simulink model "ap_12B_cocoSim_pp"  (Simulink 8.5)
settings: Solver=ode3  StartTime=0.0  StopTime=100  FixedStep=Ts  RelTol=1e-3
undefined symbols (not defined in the file): beaver_b, beaver_c, beaver_mass, beaver_S, Cl0, Cl_alpha2_dpt, Cl_beta, Cl_da, Cl_da_alpha, Cl_dr, Cl_p, Cl_r, Cm0, Cm_alpha, Cm_alpha2, Cm_beta2, Cm_de, Cm_df, Cm_dpt, Cm_q, Cm_r, Cn0, Cn_beta, Cn_beta3, Cn_da, Cn_dpt3, Cn_dr, Cn_p, Cn_q, Cn_r, Cx0, Cx_alpha, Cx_alpha2, Cx_alpha3, Cx_df, Cx_df_alpha, Cx_dpt, Cx_dpt2_alpha, Cx_dr, Cx_q, Cy0, Cy_beta, Cy_da, Cy_dr, Cy_dr_alpha, Cy_p, Cy_r, Cz0, Cz_alpha, Cz_alpha3, Cz_de, Cz_de_beta, Cz_df, Cz_df_alpha, Cz_dpt, Cz_q, d2r, fin_act_1, fin_act_2, fin_act_3 ... (+23)
libraries: simulink x12, aerolibtransform2 x9, aerolibutil x7, aerolibasang x7, aerolibadynsys x3, aerolib6dofsys x2, aerolib6dof2 x1
(part 3 of 3)

== system ap_12B_cocoSim_pp/Autopilot/Pitch_Autopilot/Altitude Mode/Lookup Table_pp/Interpolate5 ==
  InportIn : Inport
  InportIdx1 : Inport  Port=2
  InportIdx2 : Inport  Port=3
  InportData1 : Inport  Port=4
  InportData2 : Inport  Port=5
  Interpolate : Product  Inputs=*/*  SaturateOnIntegerOverflow=on  RndMeth=Zero  InputSameDT=on  OutDataTypeStr=Inherit: Same as first input
  Sum1 : Sum  Inputs=+-  SaturateOnIntegerOverflow=on  InputSameDT=on  OutDataTypeStr=Inherit: Same as first input
  Sum2 : Sum  Inputs=-+  SaturateOnIntegerOverflow=on  InputSameDT=on  OutDataTypeStr=Inherit: Same as first input
  Sum3 : Sum  Inputs=-+  SaturateOnIntegerOverflow=on  InputSameDT=on  OutDataTypeStr=Inherit: Same as first input
  Sum4 : Sum  SaturateOnIntegerOverflow=on  InputSameDT=on  OutDataTypeStr=Inherit: Same as first input
  Out : Outport
  wires:
  InportIn/1 -> Sum1/1
  InportIdx1/1 -> Sum1/2, Sum2/1
  InportIdx2/1 -> Sum2/2
  InportData1/1 -> Sum3/1, Sum4/2
  InportData2/1 -> Sum3/2
  Sum1/1 -> Interpolate/1
  Sum2/1 -> Interpolate/2
  Sum3/1 -> Interpolate/3
  Interpolate/1 -> Sum4/1
  Sum4/1 -> Out/1

== system ap_12B_cocoSim_pp/Autopilot/Pitch_Autopilot/Altitude Mode/Lookup Table_pp/Interpolate6 ==
  InportIn : Inport
  InportIdx1 : Inport  Port=2
  InportIdx2 : Inport  Port=3
  InportData1 : Inport  Port=4
  InportData2 : Inport  Port=5
  Interpolate : Product  Inputs=*/*  SaturateOnIntegerOverflow=on  RndMeth=Zero  InputSameDT=on  OutDataTypeStr=Inherit: Same as first input
  Sum1 : Sum  Inputs=+-  SaturateOnIntegerOverflow=on  InputSameDT=on  OutDataTypeStr=Inherit: Same as first input
  Sum2 : Sum  Inputs=-+  SaturateOnIntegerOverflow=on  InputSameDT=on  OutDataTypeStr=Inherit: Same as first input
  Sum3 : Sum  Inputs=-+  SaturateOnIntegerOverflow=on  InputSameDT=on  OutDataTypeStr=Inherit: Same as first input
  Sum4 : Sum  SaturateOnIntegerOverflow=on  InputSameDT=on  OutDataTypeStr=Inherit: Same as first input
  Out : Outport
  wires:
  InportIn/1 -> Sum1/1
  InportIdx1/1 -> Sum1/2, Sum2/1
  InportIdx2/1 -> Sum2/2
  InportData1/1 -> Sum3/1, Sum4/2
  InportData2/1 -> Sum3/2
  Sum1/1 -> Interpolate/1
  Sum2/1 -> Interpolate/2
  Sum3/1 -> Interpolate/3
  Interpolate/1 -> Sum4/1
  Sum4/1 -> Out/1

== system ap_12B_cocoSim_pp/Autopilot/Pitch_Autopilot/Altitude Mode/Lookup Table_pp/Interpolate7 ==
  InportIn : Inport
  InportIdx1 : Inport  Port=2
  InportIdx2 : Inport  Port=3
  InportData1 : Inport  Port=4
  InportData2 : Inport  Port=5
  Interpolate : Product  Inputs=*/*  SaturateOnIntegerOverflow=on  RndMeth=Zero  InputSameDT=on  OutDataTypeStr=Inherit: Same as first input
  Sum1 : Sum  Inputs=+-  SaturateOnIntegerOverflow=on  InputSameDT=on  OutDataTypeStr=Inherit: Same as first input
  Sum2 : Sum  Inputs=-+  SaturateOnIntegerOverflow=on  InputSameDT=on  OutDataTypeStr=Inherit: Same as first input
  Sum3 : Sum  Inputs=-+  SaturateOnIntegerOverflow=on  InputSameDT=on  OutDataTypeStr=Inherit: Same as first input
  Sum4 : Sum  SaturateOnIntegerOverflow=on  InputSameDT=on  OutDataTypeStr=Inherit: Same as first input
  Out : Outport
  wires:
  InportIn/1 -> Sum1/1
  InportIdx1/1 -> Sum1/2, Sum2/1
  InportIdx2/1 -> Sum2/2
  InportData1/1 -> Sum3/1, Sum4/2
  InportData2/1 -> Sum3/2
  Sum1/1 -> Interpolate/1
  Sum2/1 -> Interpolate/2
  Sum3/1 -> Interpolate/3
  Interpolate/1 -> Sum4/1
  Sum4/1 -> Out/1

== system ap_12B_cocoSim_pp/DeHavilland Beaver Airframe/Aircraft Dynamics/6DoF (Quaternion)/Calculate DCM & Euler Angles/Quaternions to  Direction Cosine Matrix ==
  Quat : Inport  PortDimensions=4
  A11 : aerolibtransform2/Quaternions to  Direction Cosine Matrix/A11
  A12 : aerolibtransform2/Quaternions to  Direction Cosine Matrix/A12
  A13 : aerolibtransform2/Quaternions to  Direction Cosine Matrix/A13
  A21 : aerolibtransform2/Quaternions to  Direction Cosine Matrix/A21
  A22 : aerolibtransform2/Quaternions to  Direction Cosine Matrix/A22
  A23 : aerolibtransform2/Quaternions to  Direction Cosine Matrix/A23
  A31 : aerolibtransform2/Quaternions to  Direction Cosine Matrix/A31
  A32 : aerolibtransform2/Quaternions to  Direction Cosine Matrix/A32
  A33 : aerolibtransform2/Quaternions to  Direction Cosine Matrix/A33
  Create Transformation Matrix : aerolibutil/Create 3x3 Matrix
  Quaternion Normalize : Subsystem
  DCM : Outport  PortDimensions=[3,3]  InitialOutput=0
  wires:
  Create Transformation Matrix/1 -> DCM/1
  A11/1 -> Create Transformation Matrix/1
  A21/1 -> Create Transformation Matrix/4
  A31/1 -> Create Transformation Matrix/7
  A32/1 -> Create Transformation Matrix/8
  A13/1 -> Create Transformation Matrix/3
  A23/1 -> Create Transformation Matrix/6
  A33/1 -> Create Transformation Matrix/9
  Quat/1 -> Quaternion Normalize/1(q)
  Quaternion Normalize/1(normal(q)) -> A33/1, A32/1, A31/1, A23/1, A22/1, A21/1, A13/1, A12/1, A11/1
  A22/1 -> Create Transformation Matrix/5
  A12/1 -> Create Transformation Matrix/2

== system ap_12B_cocoSim_pp/DeHavilland Beaver Airframe/Aircraft Dynamics/6DoF (Quaternion)/Calculate DCM & Euler Angles/Quaternions to Rotation Angles (ZYX) ==
  q : Inport
  Quaternion Normalize : Subsystem
  Trigonometric Function1 : Trigonometry  Operator=atan2
  Trigonometric Function3 : Trigonometry  Operator=atan2
  Vector Concatenate : Concatenate  NumInputs=3
  fcn1 : Fcn  Expr=2*(u[2]*u[3] + u[1]*u[4])
  fcn2 : Fcn  Expr=u[1]*u[1] + u[2]*u[2] - u[3]*u[3] - u[4]*u[4]
  fcn3 : Fcn  Expr=-2*(u[2]*u[4] - u[1]*u[3])
  fcn4 : Fcn  Expr=2*(u[3]*u[4] + u[1]*u[2])
  fcn5 : Fcn  Expr=u[1]*u[1] - u[2]*u[2] - u[3]*u[3] + u[4]*u[4]
  trigFcn : Trigonometry  Operator=asin
  R1,R2,R3 : Outport
  wires:
  fcn5/1 -> Trigonometric Function3/2
  fcn4/1 -> Trigonometric Function3/1
  fcn2/1 -> Trigonometric Function1/2
  fcn3/1 -> trigFcn/1
  q/1 -> Quaternion Normalize/1(q)
  Vector Concatenate/1 -> R1,R2,R3/1
  Trigonometric Function3/1 -> Vector Concatenate/3  "r3"
  Trigonometric Function1/1 -> Vector Concatenate/1  "r1"
  Quaternion Normalize/1(normal(q)) -> fcn1/1, fcn2/1, fcn5/1, fcn4/1, fcn3/1
  trigFcn/1 -> Vector Concatenate/2  "r2"
  fcn1/1 -> Trigonometric Function1/1

== system ap_12B_cocoSim_pp/DeHavilland Beaver Airframe/Aircraft Dynamics/6DoF (Quaternion)/Calculate DCM & Euler Angles/ResetIntegratorInternal1 ==
  note: ic
  note: Level Reset Integration With Saturation
      | y(n) = y(n-1) + K*Ts*u(n-1)
  U : Inport
  R : Inport  Port=2
  IC : Inport  Port=3
  Constant : Constant  Value=1.0
  Constant1 : Constant  Value=Ts
  Product : Product  RndMeth=Zero
  Product1 : Product  RndMeth=Zero
  Saturation : Saturate  UpperLimit=20  LowerLimit=-20
  Sum3 : Sum
  Switch : Switch  Criteria=u2 ~= 0
  Switch1 : Switch  Criteria=u2 ~= 0
  X : UnitDelay  SampleTime=Ts
  Y : Outport
  wires:
  Product1/1 -> Sum3/1
  U/1 -> Product1/2
  Sum3/1 -> Switch1/3
  Product/1 -> Product1/1
  Switch/1 -> Saturation/1
  IC/1 -> Switch1/1, Switch/1
  Constant1/1 -> Product/2  "deltaT"
  Switch1/1 -> X/1
  Constant/1 -> Product/1  "gain"
  Saturation/1 -> Y/1, Sum3/2
  R/1 -> Switch1/2, Switch/2
  X/1 -> Switch/3

== system ap_12B_cocoSim_pp/DeHavilland Beaver Airframe/Aircraft Dynamics/6DoF (Quaternion)/Calculate DCM & Euler Angles/Rotation Angles to Quats (ZYX) ==
  "R1, R2, R3" : Inport
  1/2 : Gain  Gain=0.5  SaturateOnIntegerOverflow=on  OutDataTypeStr=Inherit: Same as input  ParamDataTypeStr=Inherit: Same as input
  Mux1 : Mux  Inputs=2
  Mux2 : Mux
  q0 : Fcn  Expr=u(4)*u(5)*u(6) + u(1)*u(2)*u(3)
  q1 : Fcn  Expr=u(4)*u(5)*u(3) - u(1)*u(2)*u(6)
  q2 : Fcn  Expr=u(4)*u(2)*u(6) + u(1)*u(5)*u(3)
  q3 : Fcn  Expr=u(1)*u(5)*u(6) - u(4)*u(2)*u(3)
  sincos : Trigonometry  Operator=sincos
  Quat : Outport  InitialOutput=0
  wires:
  sincos/1 -> Mux1/1
  1/2/1 -> sincos/1
  "R1, R2, R3"/1 -> 1/2/1
  sincos/2 -> Mux1/2
  Mux1/1 -> q0/1, q1/1, q2/1, q3/1
  q1/1 -> Mux2/2
  q2/1 -> Mux2/3
  q3/1 -> Mux2/4
  Mux2/1 -> Quat/1
  q0/1 -> Mux2/1

== system ap_12B_cocoSim_pp/DeHavilland Beaver Airframe/Aircraft Dynamics/6DoF (Quaternion)/Calculate DCM & Euler Angles/ic3 ==
  ic : Inport
  Constant : Constant  Value=0
  Unit Delay : UnitDelay  InitialCondition=1  SampleTime=-1
  R : Outport
  IC : Outport  Port=2
  wires:
  Constant/1 -> Unit Delay/1
  Unit Delay/1 -> R/1
  ic/1 -> IC/1

== system ap_12B_cocoSim_pp/DeHavilland Beaver Airframe/Aircraft Dynamics/6DoF (Quaternion)/Calculate DCM & Euler Angles/qd ==
  p q r : Inport
  q0 q1 q2 q3 : Inport  Port=2
  Constant : Constant
  Dot Product : DotProduct  OutDataTypeStr=Inherit: Inherit via internal rule
  High Gain Quaternion Normalization : Gain  Gain=1.0  SaturateOnIntegerOverflow=on  OutDataTypeStr=Inherit: Same as input  ParamDataTypeStr=Inherit: Same as input
  Mux1 : Mux  Inputs=[3 4 1]
  Mux2 : Mux
  Sum : Sum  Inputs=|+-  SaturateOnIntegerOverflow=on  InputSameDT=on  OutDataTypeStr=Inherit: Same as first input
  q0dot : Fcn  Expr=-0.5 * ( u[5]*u[1]+u[6]*u[2]+u[7]*u[3] ) + u[8]*u[4]
  q1dot : Fcn  Expr=0.5 * ( u[4]*u[1]+u[6]*u[3]-u[7]*u[2] ) + u[8]*u[5]
  q2dot : Fcn  Expr=0.5 * ( u[4]*u[2]+u[7]*u[1]-u[5]*u[3] ) + u[8]*u[6]
  q3dot : Fcn  Expr=0.5 * ( u[4]*u[3]+u[5]*u[2]-u[6]*u[1] ) + u[8]*u[7]
  qdot : Outport  InitialOutput=0
  wires:
  p q r/1 -> Mux1/1
  q3dot/1 -> Mux2/4
  q2dot/1 -> Mux2/3
  q1dot/1 -> Mux2/2
  Constant/1 -> Sum/1
  Mux1/1 -> q2dot/1, q3dot/1, q0dot/1, q1dot/1
  q0dot/1 -> Mux2/1
  Mux2/1 -> qdot/1
  Sum/1 -> High Gain Quaternion Normalization/1
  Dot Product/1 -> Sum/2
  High Gain Quaternion Normalization/1 -> Mux1/3
  q0 q1 q2 q3/1 -> Dot Product/1, Dot Product/2, Mux1/2

== system ap_12B_cocoSim_pp/DeHavilland Beaver Airframe/Aircraft Dynamics/6DoF (Quaternion)/Calculate omega_dot/3x3 CrossProduct ==
  A : Inport
  B : Inport  Port=2
  A_1 : InportShadow
  B_1 : InportShadow  Port=2
  Subsystem : aerolibutil/3x3 Cross Product/Subsystem
  Subsystem1 : aerolibutil/3x3 Cross Product/Subsystem1
  Sum : Sum  Inputs=+|-  SaturateOnIntegerOverflow=on  InputSameDT=on  OutDataTypeStr=Inherit: Same as first input
  C : Outport
  wires:
  Subsystem/1 -> Sum/1
  Subsystem1/1 -> Sum/2
  B/1 -> Subsystem/2
  A/1 -> Subsystem/1
  B_1/1 -> Subsystem1/2
  A_1/1 -> Subsystem1/1
  Sum/1 -> C/1

== system ap_12B_cocoSim_pp/DeHavilland Beaver Airframe/Aircraft Dynamics/Total Forces  and Moments/Actuators/sof ==
  Ac_dem : Inport
  2*zeta * wn : Gain  Gain=2.0 * z_fin* wn_fin  SaturateOnIntegerOverflow=on  OutDataTypeStr=Inherit: Same as input  ParamDataTypeStr=Inherit: Same as input
  Demand limits : Saturate  UpperLimit=fin_max  LowerLimit=fin_min
  ResetIntegratorInternal : Subsystem
  ResetIntegratorInternal1 : Subsystem
  Sum2 : Sum  Inputs=|+-  SaturateOnIntegerOverflow=on  InputSameDT=on  OutDataTypeStr=Inherit: Same as first input
  Sum3 : Sum  Inputs=|+-  SaturateOnIntegerOverflow=on  InputSameDT=on  OutDataTypeStr=Inherit: Same as first input
  ic1 : Subsystem
  ic3 : Subsystem
  rate limit*2*zeta/wn : Saturate  UpperLimit=fin_maxrate*2*z_fin/wn_fin  LowerLimit=-fin_maxrate*2*z_fin/wn_fin
  wn^2 : Gain  Gain=wn_fin* wn_fin  SaturateOnIntegerOverflow=on  OutDataTypeStr=Inherit: Same as input  ParamDataTypeStr=Inherit: Same as input
  Ac_ac : Outport  InitialOutput=0
  wires:
  ResetIntegratorInternal1/1(Y) -> Ac_ac/1, Sum3/2
  wn^2/1 -> Sum2/1
  ResetIntegratorInternal/1(Y) -> ResetIntegratorInternal1/1(U), 2*zeta * wn/1
  Sum2/1 -> ResetIntegratorInternal/1(U)
  Demand limits/1 -> Sum3/1
  rate limit*2*zeta/wn/1 -> wn^2/1
  Ac_dem/1 -> Demand limits/1
  Sum3/1 -> rate limit*2*zeta/wn/1
  2*zeta * wn/1 -> Sum2/2
  ic3/2(IC) -> ResetIntegratorInternal/3(ic)
  ic3/1(R) -> ResetIntegratorInternal/2(R)
  ic1/1(R) -> ResetIntegratorInternal1/2(R)
  ic1/2(IC) -> ResetIntegratorInternal1/3(ic)

== system ap_12B_cocoSim_pp/DeHavilland Beaver Airframe/Aircraft Dynamics/Total Forces  and Moments/Actuators/sof1 ==
  Ac_dem : Inport
  2*zeta * wn : Gain  Gain=2.0 * z_fin* wn_fin  SaturateOnIntegerOverflow=on  OutDataTypeStr=Inherit: Same as input  ParamDataTypeStr=Inherit: Same as input
  Demand limits : Saturate  UpperLimit=fin_max  LowerLimit=fin_min
  ResetIntegratorInternal : Subsystem
  ResetIntegratorInternal1 : Subsystem
  Sum2 : Sum  Inputs=|+-  SaturateOnIntegerOverflow=on  InputSameDT=on  OutDataTypeStr=Inherit: Same as first input
  Sum3 : Sum  Inputs=|+-  SaturateOnIntegerOverflow=on  InputSameDT=on  OutDataTypeStr=Inherit: Same as first input
  ic1 : Subsystem
  ic3 : Subsystem
  rate limit*2*zeta/wn : Saturate  UpperLimit=fin_maxrate*2*z_fin/wn_fin  LowerLimit=-fin_maxrate*2*z_fin/wn_fin
  wn^2 : Gain  Gain=wn_fin* wn_fin  SaturateOnIntegerOverflow=on  OutDataTypeStr=Inherit: Same as input  ParamDataTypeStr=Inherit: Same as input
  Ac_ac : Outport  InitialOutput=0
  wires:
  ic1/2(IC) -> ResetIntegratorInternal1/3(ic)
  ic1/1(R) -> ResetIntegratorInternal1/2(R)
  ic3/1(R) -> ResetIntegratorInternal/2(R)
  ic3/2(IC) -> ResetIntegratorInternal/3(ic)
  2*zeta * wn/1 -> Sum2/2
  Sum3/1 -> rate limit*2*zeta/wn/1
  Ac_dem/1 -> Demand limits/1
  rate limit*2*zeta/wn/1 -> wn^2/1
  Demand limits/1 -> Sum3/1
  Sum2/1 -> ResetIntegratorInternal/1(U)
  ResetIntegratorInternal/1(Y) -> 2*zeta * wn/1, ResetIntegratorInternal1/1(U)
  wn^2/1 -> Sum2/1
  ResetIntegratorInternal1/1(Y) -> Sum3/2, Ac_ac/1

== system ap_12B_cocoSim_pp/DeHavilland Beaver Airframe/Aircraft Dynamics/Total Forces  and Moments/Actuators/sof2 ==
  Ac_dem : Inport
  2*zeta * wn : Gain  Gain=2.0 * z_fin* wn_fin  SaturateOnIntegerOverflow=on  OutDataTypeStr=Inherit: Same as input  ParamDataTypeStr=Inherit: Same as input
  Demand limits : Saturate  UpperLimit=fin_max  LowerLimit=fin_min
  ResetIntegratorInternal : Subsystem
  ResetIntegratorInternal1 : Subsystem
  Sum2 : Sum  Inputs=|+-  SaturateOnIntegerOverflow=on  InputSameDT=on  OutDataTypeStr=Inherit: Same as first input
  Sum3 : Sum  Inputs=|+-  SaturateOnIntegerOverflow=on  InputSameDT=on  OutDataTypeStr=Inherit: Same as first input
  ic1 : Subsystem
  ic3 : Subsystem
  rate limit*2*zeta/wn : Saturate  UpperLimit=fin_maxrate*2*z_fin/wn_fin  LowerLimit=-fin_maxrate*2*z_fin/wn_fin
  wn^2 : Gain  Gain=wn_fin* wn_fin  SaturateOnIntegerOverflow=on  OutDataTypeStr=Inherit: Same as input  ParamDataTypeStr=Inherit: Same as input
  Ac_ac : Outport  InitialOutput=0
  wires:
  ResetIntegratorInternal1/1(Y) -> Ac_ac/1, Sum3/2
  wn^2/1 -> Sum2/1
  ResetIntegratorInternal/1(Y) -> ResetIntegratorInternal1/1(U), 2*zeta * wn/1
  Sum2/1 -> ResetIntegratorInternal/1(U)
  Demand limits/1 -> Sum3/1
  rate limit*2*zeta/wn/1 -> wn^2/1
  Ac_dem/1 -> Demand limits/1
  Sum3/1 -> rate limit*2*zeta/wn/1
  2*zeta * wn/1 -> Sum2/2
  ic3/2(IC) -> ResetIntegratorInternal/3(ic)
  ic3/1(R) -> ResetIntegratorInternal/2(R)
  ic1/1(R) -> ResetIntegratorInternal1/2(R)
  ic1/2(IC) -> ResetIntegratorInternal1/3(ic)

== system ap_12B_cocoSim_pp/DeHavilland Beaver Airframe/Aircraft Dynamics/Total Forces  and Moments/Aerodynamics/Actuator Increments ==
  alpha : Inport
  beta : Inport  Port=2
  Actuator Deflections : Inport  Port=3
  Aileron : Subsystem
  Elevator : Subsystem
  Flap : Subsystem
  Rudder : Subsystem
  Sum1 : Sum  SaturateOnIntegerOverflow=on
  Sum2 : Sum  SaturateOnIntegerOverflow=on
  Sum3 : Sum  SaturateOnIntegerOverflow=on
  Coefficients : Outport
  wires:
  Actuator Deflections/1 -> Flap/2(Actuators), Aileron/2(Actuators), Elevator/1(Actuators), Rudder/2(Actuators)
  alpha/1 -> Flap/1(Alpha), Rudder/1(Alpha), Aileron/1(alpha)
  beta/1 -> Elevator/2(Beta)
  Aileron/1(delCoeff) -> Sum1/1
  Elevator/1(delCoeff) -> Sum1/2
  Rudder/1(delCoeff) -> Sum2/2
  Flap/1(delCoeff) -> Sum3/2
  Sum3/1 -> Coefficients/1
  Sum1/1 -> Sum2/1
  Sum2/1 -> Sum3/1

== system ap_12B_cocoSim_pp/DeHavilland Beaver Airframe/Aircraft Dynamics/Total Forces  and Moments/Aerodynamics/Body Rate Damping ==
  V : Inport
  p,q,r : Inport  Port=2
  Demux : Demux  Outputs=3
  Product : Product  SaturateOnIntegerOverflow=on  InputSameDT=on  OutDataTypeStr=Inherit: Same as first input
  Product1 : Product  SaturateOnIntegerOverflow=on  InputSameDT=on  OutDataTypeStr=Inherit: Same as first input
  Product2 : Product  SaturateOnIntegerOverflow=on  InputSameDT=on  OutDataTypeStr=Inherit: Same as first input
  Product3 : Product  Inputs=*/  SaturateOnIntegerOverflow=on  InputSameDT=on  OutDataTypeStr=Inherit: Same as first input
  Reference Length : Gain  Gain=beaver_c  SaturateOnIntegerOverflow=on  OutDataTypeStr=Inherit: Same as input  ParamDataTypeStr=Inherit: Same as input
  Reference Span : Gain  Gain=beaver_b/2  SaturateOnIntegerOverflow=on  OutDataTypeStr=Inherit: Same as input  ParamDataTypeStr=Inherit: Same as input
  "Reference Span " : Gain  Gain=beaver_b/2  SaturateOnIntegerOverflow=on  OutDataTypeStr=Inherit: Same as input  ParamDataTypeStr=Inherit: Same as input
  Sum1 : Sum  SaturateOnIntegerOverflow=on
  Sum2 : Sum  SaturateOnIntegerOverflow=on
  p : Subsystem
  q : Subsystem
  r : Subsystem
  Coefficients : Outport
  wires:
  p/1(delCoeff) -> Product/1
  q/1(delCoeff) -> Product1/1
  p,q,r/1 -> Demux/1
  Demux/1 -> Product/2  "p"
  Demux/2 -> Product1/2  "q"
  Demux/3 -> Product2/2  "r"
  Sum1/1 -> Product3/1
  V/1 -> Product3/2
  Product3/1 -> Coefficients/1
  Product1/1 -> Reference Length/1
  Product2/1 -> "Reference Span "/1
  Product/1 -> Reference Span/1
  r/1(delCoeff) -> Product2/1
  Reference Length/1 -> Sum2/2
  "Reference Span "/1 -> Sum1/2
  Reference Span/1 -> Sum2/1
  Sum2/1 -> Sum1/1

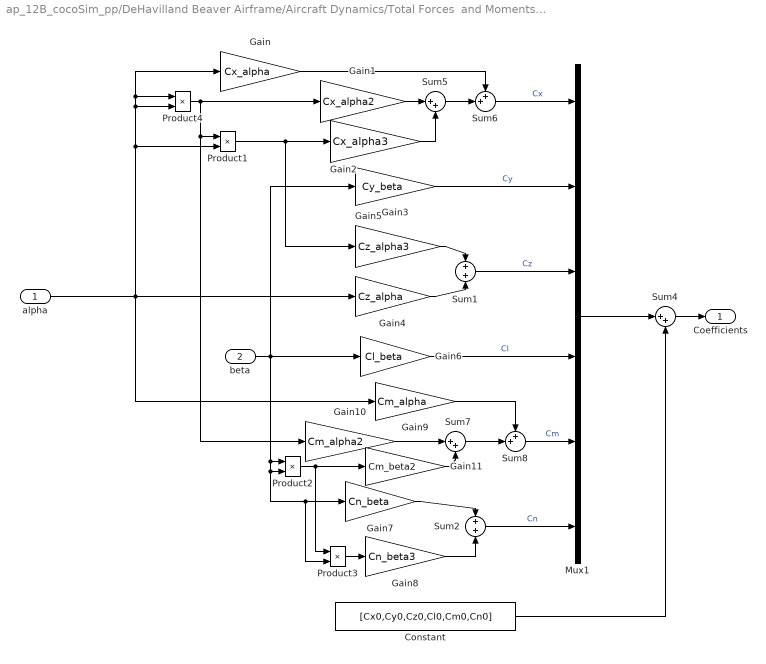
== system ap_12B_cocoSim_pp/DeHavilland Beaver Airframe/Aircraft Dynamics/Total Forces  and Moments/Aerodynamics/Datum Coefficients ==
  alpha : Inport
  beta : Inport  Port=2
  Constant : Constant  Value=[Cx0,Cy0,Cz0,Cl0,Cm0,Cn0]
  Gain : Gain  Gain=Cx_alpha  SaturateOnIntegerOverflow=on  OutDataTypeStr=Inherit: Same as input  ParamDataTypeStr=Inherit: Same as input
  Gain1 : Gain  Gain=Cx_alpha2  SaturateOnIntegerOverflow=on  OutDataTypeStr=Inherit: Same as input  ParamDataTypeStr=Inherit: Same as input
  Gain10 : Gain  Gain=Cm_alpha2  SaturateOnIntegerOverflow=on  OutDataTypeStr=Inherit: Same as input  ParamDataTypeStr=Inherit: Same as input
  Gain11 : Gain  Gain=Cm_beta2  SaturateOnIntegerOverflow=on  OutDataTypeStr=Inherit: Same as input  ParamDataTypeStr=Inherit: Same as input
  Gain2 : Gain  Gain=Cx_alpha3  SaturateOnIntegerOverflow=on  OutDataTypeStr=Inherit: Same as input  ParamDataTypeStr=Inherit: Same as input
  Gain3 : Gain  Gain=Cy_beta  SaturateOnIntegerOverflow=on  OutDataTypeStr=Inherit: Same as input  ParamDataTypeStr=Inherit: Same as input
  Gain4 : Gain  Gain=Cz_alpha  SaturateOnIntegerOverflow=on  OutDataTypeStr=Inherit: Same as input  ParamDataTypeStr=Inherit: Same as input
  Gain5 : Gain  Gain=Cz_alpha3  SaturateOnIntegerOverflow=on  OutDataTypeStr=Inherit: Same as input  ParamDataTypeStr=Inherit: Same as input
  Gain6 : Gain  Gain=Cl_beta  SaturateOnIntegerOverflow=on  OutDataTypeStr=Inherit: Same as input  ParamDataTypeStr=Inherit: Same as input
  Gain7 : Gain  Gain=Cn_beta  SaturateOnIntegerOverflow=on  OutDataTypeStr=Inherit: Same as input  ParamDataTypeStr=Inherit: Same as input
  Gain8 : Gain  Gain=Cn_beta3  SaturateOnIntegerOverflow=on  OutDataTypeStr=Inherit: Same as input  ParamDataTypeStr=Inherit: Same as input
  Gain9 : Gain  Gain=Cm_alpha  SaturateOnIntegerOverflow=on  OutDataTypeStr=Inherit: Same as input  ParamDataTypeStr=Inherit: Same as input
  Mux1 : Mux  Inputs=6
  Product{1..4} (4 alike) : Product  SaturateOnIntegerOverflow=on  InputSameDT=on  OutDataTypeStr=Inherit: Same as first input
  Sum1 : Sum  SaturateOnIntegerOverflow=on
  Sum2 : Sum  SaturateOnIntegerOverflow=on
  Sum4 : Sum  Inputs=|++  SaturateOnIntegerOverflow=on
  Sum5 : Sum  Inputs=|++  SaturateOnIntegerOverflow=on
  Sum6 : Sum  Inputs=++|  SaturateOnIntegerOverflow=on
  Sum7 : Sum  Inputs=|++  SaturateOnIntegerOverflow=on
  Sum8 : Sum  Inputs=++|  SaturateOnIntegerOverflow=on
  Coefficients : Outport
  wires:
  Constant/1 -> Sum4/2
  Sum4/1 -> Coefficients/1
  Mux1/1 -> Sum4/1
  Gain10/1 -> Sum7/1
  Product2/1 -> Product3/1, Gain11/1
  Gain11/1 -> Sum7/2
  Gain9/1 -> Sum8/1
  Sum8/1 -> Mux1/5  "Cm"
  Product3/1 -> Gain8/1
  Gain8/1 -> Sum2/2
  Gain7/1 -> Sum2/1
  Gain5/1 -> Sum1/1
  Gain4/1 -> Sum1/2
  Product1/1 -> Gain5/1, Gain2/1
  Product4/1 -> Product1/1, Gain10/1, Gain1/1
  Gain/1 -> Sum6/1
  Sum2/1 -> Mux1/6  "Cn"
  Sum6/1 -> Mux1/1  "Cx"
  Sum1/1 -> Mux1/3  "Cz"
  Gain3/1 -> Mux1/2  "Cy"
  Gain6/1 -> Mux1/4  "Cl"
  alpha/1 -> Product1/2, Product4/2, Product4/1, Gain/1, Gain9/1, Gain4/1
  beta/1 -> Gain6/1, Gain3/1, Product3/2, Gain7/1, Product2/2, Product2/1
  Gain1/1 -> Sum5/1
  Gain2/1 -> Sum5/2
  Sum5/1 -> Sum6/2
  Sum7/1 -> Sum8/2

== system ap_12B_cocoSim_pp/DeHavilland Beaver Airframe/Aircraft Dynamics/Total Forces  and Moments/Engine /eng ==
  note: dpt
  dpt : Inport
  alpha : Inport  Port=2
  Constant : Constant  Value=0
  Gain1 : Gain  Gain=Cn_dpt3  SaturateOnIntegerOverflow=on  OutDataTypeStr=Inherit: Same as input  ParamDataTypeStr=Inherit: Same as input
  Gain2 : Gain  Gain=Cm_dpt  SaturateOnIntegerOverflow=on  OutDataTypeStr=Inherit: Same as input  ParamDataTypeStr=Inherit: Same as input
  Gain3 : Gain  Gain=Cl_alpha2_dpt  SaturateOnIntegerOverflow=on  OutDataTypeStr=Inherit: Same as input  ParamDataTypeStr=Inherit: Same as input
  Gain4 : Gain  Gain=Cz_dpt  SaturateOnIntegerOverflow=on  OutDataTypeStr=Inherit: Same as input  ParamDataTypeStr=Inherit: Same as input
  Gain5 : Gain  Gain=Cx_dpt  SaturateOnIntegerOverflow=on  OutDataTypeStr=Inherit: Same as input  ParamDataTypeStr=Inherit: Same as input
  Gain6 : Gain  Gain=Cx_dpt2_alpha  SaturateOnIntegerOverflow=on  OutDataTypeStr=Inherit: Same as input  ParamDataTypeStr=Inherit: Same as input
  Mux2 : Mux  Inputs=6
  Product{,1..4,6} (6 alike) : Product  SaturateOnIntegerOverflow=on  OutDataTypeStr=Inherit: Same as first input
  Sum : Sum  Inputs=|++  SaturateOnIntegerOverflow=on
  Cprop : Outport
  wires:
  Sum/1 -> Mux2/1
  Gain6/1 -> Sum/2
  Gain5/1 -> Sum/1
  Constant/1 -> Mux2/2
  Gain4/1 -> Mux2/3
  Gain3/1 -> Mux2/4
  Gain2/1 -> Mux2/5
  Gain1/1 -> Mux2/6
  Product4/1 -> Gain3/1
  Product2/1 -> Gain6/1
  dpt/1 -> Gain5/1, Product/1, Product/2, Product6/2, Product1/2, Product1/1, Gain2/1, Gain4/1, Product4/2
  alpha/1 -> Product2/2, Product3/1, Product3/2
  Mux2/1 -> Cprop/1  "Cprop"
  Product/1 -> Product2/1
  Product3/1 -> Product4/1
  Product1/1 -> Product6/1
  Product6/1 -> Gain1/1

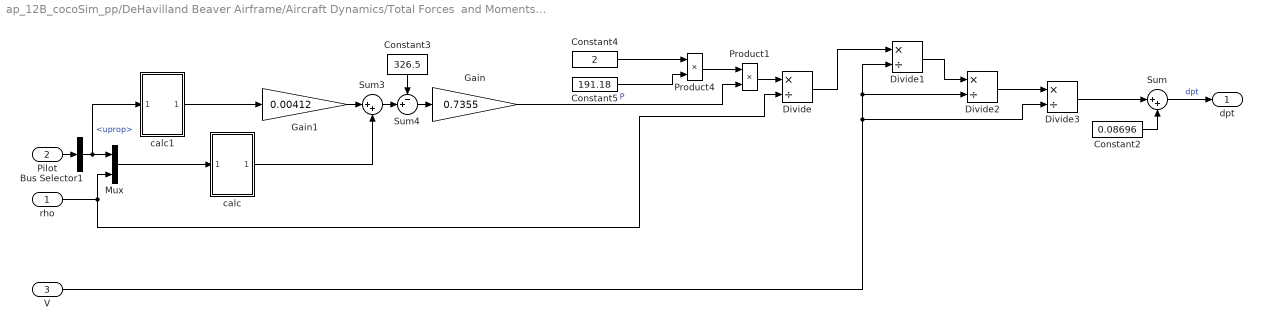
== system ap_12B_cocoSim_pp/DeHavilland Beaver Airframe/Aircraft Dynamics/Total Forces  and Moments/Engine /pow ==
  rho : Inport
  Pilot : Inport  Port=2
  V : Inport  Port=3
  Bus Selector1 : BusSelector  OutputSignals=uprop
  Constant2 : Constant  Value=0.08696
  Constant3 : Constant  Value=326.5
  Constant4 : Constant  Value=2
  Constant5 : Constant  Value=191.18
  Divide{,1..3} (4 alike) : Product  Inputs=*/
  Gain : Gain  Gain=0.7355  SaturateOnIntegerOverflow=on  OutDataTypeStr=Inherit: Same as input  ParamDataTypeStr=Inherit: Same as input
  Gain1 : Gain  Gain=0.00412  SaturateOnIntegerOverflow=on  OutDataTypeStr=Inherit: Same as input  ParamDataTypeStr=Inherit: Same as input
  Mux : Mux  Inputs=2
  Product1 : Product  SaturateOnIntegerOverflow=on  OutDataTypeStr=Inherit: Same as first input
  Product4 : Product  SaturateOnIntegerOverflow=on  OutDataTypeStr=Inherit: Same as first input
  Sum : Sum  Inputs=|++  SaturateOnIntegerOverflow=on
  Sum3 : Sum  Inputs=|++  SaturateOnIntegerOverflow=on
  Sum4 : Sum  Inputs=-+|  SaturateOnIntegerOverflow=on
  calc : Subsystem
  calc1 : Subsystem
  dpt : Outport
  wires:
  calc/1(Out1) -> Sum3/2
  Constant3/1 -> Sum4/1
  Gain1/1 -> Sum3/1
  rho/1 -> Divide/2, Mux/2
  Sum/1 -> dpt/1  "dpt"
  V/1 -> Divide3/2, Divide1/2, Divide2/2
  Bus Selector1/1 -> calc1/1(In1), Mux/1  "<uprop>"
  Divide3/1 -> Sum/1
  Constant2/1 -> Sum/2
  Pilot/1 -> Bus Selector1/1
  Sum4/1 -> Gain/1
  Sum3/1 -> Sum4/2
  Mux/1 -> calc/1(In1)
  calc1/1(Out1) -> Gain1/1
  Constant4/1 -> Product4/1
  Constant5/1 -> Product4/2
  Product4/1 -> Product1/1
  Gain/1 -> Product1/2  "P"
  Product1/1 -> Divide/1
  Divide/1 -> Divide1/1
  Divide1/1 -> Divide2/1
  Divide2/1 -> Divide3/1

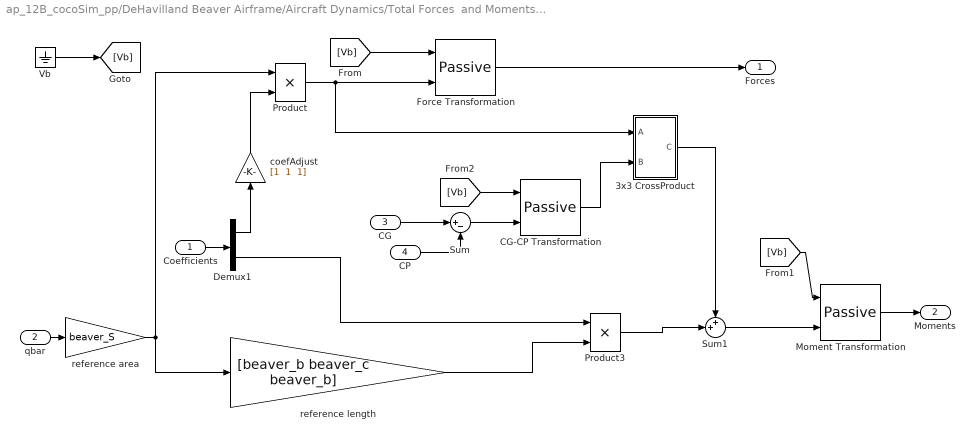
== system ap_12B_cocoSim_pp/DeHavilland Beaver Airframe/Aircraft Dynamics/Total Forces  and Moments/Forces and Moments/Aero F&M ==
  Coefficients : Inport
  qbar : Inport  Port=2
  CG : Inport  Port=3
  CP : Inport  Port=4
  3x3 CrossProduct : Subsystem
  CG-CP Transformation : aerolibadynsys/Passive  SystemSampleTime=-1
  Demux1 : Demux  Outputs=[3,3]
  Force Transformation : aerolibadynsys/Passive  SystemSampleTime=-1
  Moment Transformation : aerolibadynsys/Passive  SystemSampleTime=-1
  Product : Product  SaturateOnIntegerOverflow=on  InputSameDT=on  OutDataTypeStr=Inherit: Same as first input
  Product3 : Product  SaturateOnIntegerOverflow=on  InputSameDT=on  OutDataTypeStr=Inherit: Same as first input
  Sum : Sum  Inputs=|+-  SaturateOnIntegerOverflow=on
  Sum1 : Sum  Inputs=++|  SaturateOnIntegerOverflow=on  InputSameDT=on  OutDataTypeStr=Inherit: Same as first input
  Vb : Ground
  coefAdjust : Gain  Gain="[1  1  1]"
  reference area : Gain  Gain=beaver_S  SaturateOnIntegerOverflow=on  OutDataTypeStr=Inherit: Same as input  ParamDataTypeStr=Inherit: Same as input
  reference length : Gain  Gain=[beaver_b beaver_c beaver_b]  SaturateOnIntegerOverflow=on  OutDataTypeStr=Inherit: Same as input  ParamDataTypeStr=Inherit: Same as input
  Forces : Outport
  Moments : Outport  Port=2
  wires:
  [Vb] -> Force Transformation/1
  CP/1 -> Sum/2
  reference length/1 -> Product3/2
  Demux1/2 -> Product3/1
  qbar/1 -> reference area/1
  coefAdjust/1 -> Product/2
  Force Transformation/1 -> Forces/1
  Demux1/1 -> coefAdjust/1
  Coefficients/1 -> Demux1/1
  [Vb] -> Moment Transformation/1
  [Vb] -> CG-CP Transformation/1
  CG-CP Transformation/1 -> 3x3 CrossProduct/2(B)
  Product3/1 -> Sum1/2
  Vb/1 -> [Vb]
  reference area/1 -> reference length/1, Product/1
  Moment Transformation/1 -> Moments/1
  Product/1 -> 3x3 CrossProduct/1(A), Force Transformation/2
  Sum/1 -> CG-CP Transformation/2
  Sum1/1 -> Moment Transformation/2
  3x3 CrossProduct/1(C) -> Sum1/1
  CG/1 -> Sum/1

== system ap_12B_cocoSim_pp/DeHavilland Beaver Airframe/Aircraft Dynamics/6DoF (Quaternion)/Calculate DCM & Euler Angles/Quaternions to  Direction Cosine Matrix/Quaternion Normalize ==
  q : Inport
  Demux : Demux
  Mux : Mux
  Product{,1..3} (4 alike) : Product  Inputs=*/
  Quaternion Modulus : Subsystem
  normal(q) : Outport
  wires:
  Product3/1 -> Mux/4
  Product1/1 -> Mux/2
  Demux/1 -> Product/1
  Quaternion Modulus/1(|q|) -> Product1/2, Product/2, Product2/2, Product3/2
  Mux/1 -> normal(q)/1
  q/1 -> Quaternion Modulus/1(q), Demux/1
  Product/1 -> Mux/1
  Demux/3 -> Product2/1
  Demux/4 -> Product3/1
  Product2/1 -> Mux/3
  Demux/2 -> Product1/1

== system ap_12B_cocoSim_pp/DeHavilland Beaver Airframe/Aircraft Dynamics/6DoF (Quaternion)/Calculate DCM & Euler Angles/Quaternions to Rotation Angles (ZYX)/Quaternion Normalize ==
  q : Inport
  Demux : Demux
  Mux : Mux
  Product{,1..3} (4 alike) : Product  Inputs=*/
  Quaternion Modulus : Subsystem
  normal(q) : Outport
  wires:
  Product3/1 -> Mux/4
  Product1/1 -> Mux/2
  Demux/1 -> Product/1
  Quaternion Modulus/1(|q|) -> Product1/2, Product/2, Product2/2, Product3/2
  Mux/1 -> normal(q)/1
  q/1 -> Quaternion Modulus/1(q), Demux/1
  Product/1 -> Mux/1
  Demux/3 -> Product2/1
  Demux/4 -> Product3/1
  Product2/1 -> Mux/3
  Demux/2 -> Product1/1

== system ap_12B_cocoSim_pp/DeHavilland Beaver Airframe/Aircraft Dynamics/Total Forces  and Moments/Actuators/sof/ResetIntegratorInternal ==
  note: ic
  note: Level Reset Integration With Saturation
      | y(n) = y(n-1) + K*Ts*u(n-1)
  U : Inport
  R : Inport  Port=2
  ic : Inport  Port=3
  Constant : Constant  Value=1.0
  Constant1 : Constant  Value=Ts
  Product : Product  RndMeth=Zero
  Product1 : Product  RndMeth=Zero
  Sum3 : Sum
  Switch : Switch  Criteria=u2 ~= 0
  Switch1 : Switch  Criteria=u2 ~= 0
  X : UnitDelay  SampleTime=Ts
  Y : Outport
  wires:
  Product1/1 -> Sum3/1
  U/1 -> Product1/2
  Sum3/1 -> Switch1/3
  Product/1 -> Product1/1
  ic/1 -> Switch1/1, Switch/1
  Constant1/1 -> Product/2  "deltaT"
  Switch1/1 -> X/1
  Constant/1 -> Product/1  "gain"
  Switch/1 -> Y/1, Sum3/2
  R/1 -> Switch1/2, Switch/2
  X/1 -> Switch/3

== system ap_12B_cocoSim_pp/DeHavilland Beaver Airframe/Aircraft Dynamics/Total Forces  and Moments/Actuators/sof/ResetIntegratorInternal1 ==
  note: Level Reset Integration With Saturation
      | y(n) = y(n-1) + K*Ts*u(n-1)
  note: ic
  U : Inport
  R : Inport  Port=2
  ic : Inport  Port=3
  Constant : Constant  Value=1.0
  Constant1 : Constant  Value=Ts
  Product : Product  RndMeth=Zero
  Product1 : Product  RndMeth=Zero
  Saturation : Saturate  UpperLimit=fin_max  LowerLimit=fin_min
  Sum3 : Sum
  Switch : Switch  Criteria=u2 ~= 0
  Switch1 : Switch  Criteria=u2 ~= 0
  X : UnitDelay  SampleTime=Ts
  Y : Outport
  wires:
  X/1 -> Switch/3
  R/1 -> Switch/2, Switch1/2
  Saturation/1 -> Sum3/2, Y/1
  Constant/1 -> Product/1  "gain"
  Switch1/1 -> X/1
  Constant1/1 -> Product/2  "deltaT"
  ic/1 -> Switch/1, Switch1/1
  Switch/1 -> Saturation/1
  Product/1 -> Product1/1
  Sum3/1 -> Switch1/3
  U/1 -> Product1/2
  Product1/1 -> Sum3/1

== system ap_12B_cocoSim_pp/DeHavilland Beaver Airframe/Aircraft Dynamics/Total Forces  and Moments/Actuators/sof/ic1 ==
  Constant : Constant  Value=0
  Constant1 : Constant  Value=fin_act_1
  Unit Delay : UnitDelay  InitialCondition=1  SampleTime=-1
  R : Outport
  IC : Outport  Port=2
  wires:
  Constant1/1 -> IC/1
  Unit Delay/1 -> R/1
  Constant/1 -> Unit Delay/1

== system ap_12B_cocoSim_pp/DeHavilland Beaver Airframe/Aircraft Dynamics/Total Forces  and Moments/Actuators/sof/ic3 ==
  Constant : Constant  Value=0
  Constant1 : Constant  Value=0.0
  Unit Delay : UnitDelay  InitialCondition=1  SampleTime=-1
  R : Outport
  IC : Outport  Port=2
  wires:
  Constant/1 -> Unit Delay/1
  Unit Delay/1 -> R/1
  Constant1/1 -> IC/1

== system ap_12B_cocoSim_pp/DeHavilland Beaver Airframe/Aircraft Dynamics/Total Forces  and Moments/Actuators/sof1/ResetIntegratorInternal ==
  note: Level Reset Integration With Saturation
      | y(n) = y(n-1) + K*Ts*u(n-1)
  note: ic
  U : Inport
  R : Inport  Port=2
  ic : Inport  Port=3
  Constant : Constant  Value=1.0
  Constant1 : Constant  Value=Ts
  Product : Product  RndMeth=Zero
  Product1 : Product  RndMeth=Zero
  Sum3 : Sum
  Switch : Switch  Criteria=u2 ~= 0
  Switch1 : Switch  Criteria=u2 ~= 0
  X : UnitDelay  SampleTime=Ts
  Y : Outport
  wires:
  X/1 -> Switch/3
  R/1 -> Switch/2, Switch1/2
  Switch/1 -> Sum3/2, Y/1
  Constant/1 -> Product/1  "gain"
  Switch1/1 -> X/1
  Constant1/1 -> Product/2  "deltaT"
  ic/1 -> Switch/1, Switch1/1
  Product/1 -> Product1/1
  Sum3/1 -> Switch1/3
  U/1 -> Product1/2
  Product1/1 -> Sum3/1

== system ap_12B_cocoSim_pp/DeHavilland Beaver Airframe/Aircraft Dynamics/Total Forces  and Moments/Actuators/sof1/ResetIntegratorInternal1 ==
  note: ic
  note: Level Reset Integration With Saturation
      | y(n) = y(n-1) + K*Ts*u(n-1)
  U : Inport
  R : Inport  Port=2
  ic : Inport  Port=3
  Constant : Constant  Value=1.0
  Constant1 : Constant  Value=Ts
  Product : Product  RndMeth=Zero
  Product1 : Product  RndMeth=Zero
  Saturation : Saturate  UpperLimit=fin_max  LowerLimit=fin_min
  Sum3 : Sum
  Switch : Switch  Criteria=u2 ~= 0
  Switch1 : Switch  Criteria=u2 ~= 0
  X : UnitDelay  SampleTime=Ts
  Y : Outport
  wires:
  Product1/1 -> Sum3/1
  U/1 -> Product1/2
  Sum3/1 -> Switch1/3
  Product/1 -> Product1/1
  Switch/1 -> Saturation/1
  ic/1 -> Switch1/1, Switch/1
  Constant1/1 -> Product/2  "deltaT"
  Switch1/1 -> X/1
  Constant/1 -> Product/1  "gain"
  Saturation/1 -> Y/1, Sum3/2
  R/1 -> Switch1/2, Switch/2
  X/1 -> Switch/3

== system ap_12B_cocoSim_pp/DeHavilland Beaver Airframe/Aircraft Dynamics/Total Forces  and Moments/Actuators/sof1/ic1 ==
  Constant : Constant  Value=0
  Constant1 : Constant  Value=fin_act_2
  Unit Delay : UnitDelay  InitialCondition=1  SampleTime=-1
  R : Outport
  IC : Outport  Port=2
  wires:
  Constant/1 -> Unit Delay/1
  Unit Delay/1 -> R/1
  Constant1/1 -> IC/1

== system ap_12B_cocoSim_pp/DeHavilland Beaver Airframe/Aircraft Dynamics/Total Forces  and Moments/Actuators/sof1/ic3 ==
  Constant : Constant  Value=0
  Constant1 : Constant  Value=0.0
  Unit Delay : UnitDelay  InitialCondition=1  SampleTime=-1
  R : Outport
  IC : Outport  Port=2
  wires:
  Constant1/1 -> IC/1
  Unit Delay/1 -> R/1
  Constant/1 -> Unit Delay/1

== system ap_12B_cocoSim_pp/DeHavilland Beaver Airframe/Aircraft Dynamics/Total Forces  and Moments/Actuators/sof2/ResetIntegratorInternal ==
  note: ic
  note: Level Reset Integration With Saturation
      | y(n) = y(n-1) + K*Ts*u(n-1)
  U : Inport
  R : Inport  Port=2
  ic : Inport  Port=3
  Constant : Constant  Value=1.0
  Constant1 : Constant  Value=Ts
  Product : Product  RndMeth=Zero
  Product1 : Product  RndMeth=Zero
  Sum3 : Sum
  Switch : Switch  Criteria=u2 ~= 0
  Switch1 : Switch  Criteria=u2 ~= 0
  X : UnitDelay  SampleTime=Ts
  Y : Outport
  wires:
  Product1/1 -> Sum3/1
  U/1 -> Product1/2
  Sum3/1 -> Switch1/3
  Product/1 -> Product1/1
  ic/1 -> Switch1/1, Switch/1
  Constant1/1 -> Product/2  "deltaT"
  Switch1/1 -> X/1
  Constant/1 -> Product/1  "gain"
  Switch/1 -> Y/1, Sum3/2
  R/1 -> Switch1/2, Switch/2
  X/1 -> Switch/3

== system ap_12B_cocoSim_pp/DeHavilland Beaver Airframe/Aircraft Dynamics/Total Forces  and Moments/Actuators/sof2/ResetIntegratorInternal1 ==
  note: Level Reset Integration With Saturation
      | y(n) = y(n-1) + K*Ts*u(n-1)
  note: ic
  U : Inport
  R : Inport  Port=2
  ic : Inport  Port=3
  Constant : Constant  Value=1.0
  Constant1 : Constant  Value=Ts
  Product : Product  RndMeth=Zero
  Product1 : Product  RndMeth=Zero
  Saturation : Saturate  UpperLimit=fin_max  LowerLimit=fin_min
  Sum3 : Sum
  Switch : Switch  Criteria=u2 ~= 0
  Switch1 : Switch  Criteria=u2 ~= 0
  X : UnitDelay  SampleTime=Ts
  Y : Outport
  wires:
  X/1 -> Switch/3
  R/1 -> Switch/2, Switch1/2
  Saturation/1 -> Sum3/2, Y/1
  Constant/1 -> Product/1  "gain"
  Switch1/1 -> X/1
  Constant1/1 -> Product/2  "deltaT"
  ic/1 -> Switch/1, Switch1/1
  Switch/1 -> Saturation/1
  Product/1 -> Product1/1
  Sum3/1 -> Switch1/3
  U/1 -> Product1/2
  Product1/1 -> Sum3/1

== system ap_12B_cocoSim_pp/DeHavilland Beaver Airframe/Aircraft Dynamics/Total Forces  and Moments/Actuators/sof2/ic1 ==
  Constant : Constant  Value=0
  Constant1 : Constant  Value=fin_act_3
  Unit Delay : UnitDelay  InitialCondition=1  SampleTime=-1
  R : Outport
  IC : Outport  Port=2
  wires:
  Constant1/1 -> IC/1
  Unit Delay/1 -> R/1
  Constant/1 -> Unit Delay/1

== system ap_12B_cocoSim_pp/DeHavilland Beaver Airframe/Aircraft Dynamics/Total Forces  and Moments/Actuators/sof2/ic3 ==
  Constant : Constant  Value=0
  Constant1 : Constant  Value=0.0
  Unit Delay : UnitDelay  InitialCondition=1  SampleTime=-1
  R : Outport
  IC : Outport  Port=2
  wires:
  Constant/1 -> Unit Delay/1
  Unit Delay/1 -> R/1
  Constant1/1 -> IC/1

== system ap_12B_cocoSim_pp/DeHavilland Beaver Airframe/Aircraft Dynamics/Total Forces  and Moments/Aerodynamics/Actuator Increments/Aileron ==
  alpha : Inport
  Actuators : Inport  Port=2
  Gain1 : Gain  Gain=0  SaturateOnIntegerOverflow=on  OutDataTypeStr=Inherit: Same as input  ParamDataTypeStr=Inherit: Same as input
  Gain2 : Gain  Gain=Cy_da  SaturateOnIntegerOverflow=on  OutDataTypeStr=Inherit: Same as input  ParamDataTypeStr=Inherit: Same as input
  Gain3 : Gain  Gain=0  SaturateOnIntegerOverflow=on  OutDataTypeStr=Inherit: Same as input  ParamDataTypeStr=Inherit: Same as input
  Gain4 : Gain  Gain=Cn_da  SaturateOnIntegerOverflow=on  OutDataTypeStr=Inherit: Same as input  ParamDataTypeStr=Inherit: Same as input
  Gain5 : Gain  Gain=0  SaturateOnIntegerOverflow=on  OutDataTypeStr=Inherit: Same as input  ParamDataTypeStr=Inherit: Same as input
  Gain6 : Gain  Gain=Cl_da  SaturateOnIntegerOverflow=on  OutDataTypeStr=Inherit: Same as input  ParamDataTypeStr=Inherit: Same as input
  Gain7 : Gain  Gain=Cl_da_alpha  SaturateOnIntegerOverflow=on  OutDataTypeStr=Inherit: Same as input  ParamDataTypeStr=Inherit: Same as input
  Mux1 : Mux  Inputs=6
  Product4 : Product  SaturateOnIntegerOverflow=on  InputSameDT=on  OutDataTypeStr=Inherit: Same as first input
  Selector1 : Selector  InputPortWidth=4  Indices=2
  Sum1 : Sum  Inputs=++|  SaturateOnIntegerOverflow=on
  delCoeff : Outport
  wires:
  Gain6/1 -> Sum1/1
  Sum1/1 -> Mux1/4
  Gain7/1 -> Sum1/2
  Product4/1 -> Gain7/1
  Gain1/1 -> Mux1/1  "Cx"
  alpha/1 -> Product4/2
  Actuators/1 -> Selector1/1
  Mux1/1 -> delCoeff/1
  Gain2/1 -> Mux1/2  "Cy"
  Gain3/1 -> Mux1/3  "Cz"
  Gain5/1 -> Mux1/5  "Cm"
  Gain4/1 -> Mux1/6
  Selector1/1 -> Gain1/1, Gain2/1, Gain3/1, Gain6/1, Product4/1, Gain5/1, Gain4/1

== system ap_12B_cocoSim_pp/DeHavilland Beaver Airframe/Aircraft Dynamics/Total Forces  and Moments/Aerodynamics/Actuator Increments/Elevator ==
  Actuators : Inport
  Beta : Inport  Port=2
  Constant1 : Constant  Value=0
  Gain1 : Gain  Gain=Cz_de  SaturateOnIntegerOverflow=on  OutDataTypeStr=Inherit: Same as input  ParamDataTypeStr=Inherit: Same as input
  Gain2 : Gain  Gain=Cz_de_beta  SaturateOnIntegerOverflow=on  OutDataTypeStr=Inherit: Same as input  ParamDataTypeStr=Inherit: Same as input
  Gain3 : Gain  Gain=Cm_de  SaturateOnIntegerOverflow=on  OutDataTypeStr=Inherit: Same as input  ParamDataTypeStr=Inherit: Same as input
  Mux1 : Mux  Inputs=6
  Product1 : Product  SaturateOnIntegerOverflow=on  InputSameDT=on  OutDataTypeStr=Inherit: Same as first input
  Product2 : Product  SaturateOnIntegerOverflow=on  InputSameDT=on  OutDataTypeStr=Inherit: Same as first input
  Selector1 : Selector  InputPortWidth=4
  Sum1 : Sum  SaturateOnIntegerOverflow=on
  delCoeff : Outport
  wires:
  Gain3/1 -> Mux1/5
  Gain1/1 -> Sum1/2
  Gain2/1 -> Sum1/1
  Sum1/1 -> Mux1/3
  Product2/1 -> Gain2/1
  Beta/1 -> Product1/2, Product1/1
  Mux1/1 -> delCoeff/1
  Selector1/1 -> Gain3/1, Product2/2, Gain1/1
  Constant1/1 -> Mux1/1, Mux1/2, Mux1/4, Mux1/6
  Actuators/1 -> Selector1/1
  Product1/1 -> Product2/1

== system ap_12B_cocoSim_pp/DeHavilland Beaver Airframe/Aircraft Dynamics/Total Forces  and Moments/Aerodynamics/Actuator Increments/Flap ==
  Alpha : Inport
  Actuators : Inport  Port=2
  Constant1 : Constant  Value=0
  Constant2 : Constant  Value=0
  Constant3 : Constant  Value=0
  Gain1 : Gain  Gain=Cx_df  SaturateOnIntegerOverflow=on  OutDataTypeStr=Inherit: Same as input  ParamDataTypeStr=Inherit: Same as input
  Gain2 : Gain  Gain=Cx_df_alpha  SaturateOnIntegerOverflow=on  OutDataTypeStr=Inherit: Same as input  ParamDataTypeStr=Inherit: Same as input
  Gain3 : Gain  Gain=Cz_df  SaturateOnIntegerOverflow=on  OutDataTypeStr=Inherit: Same as input  ParamDataTypeStr=Inherit: Same as input
  Gain4 : Gain  Gain=Cz_df_alpha  SaturateOnIntegerOverflow=on  OutDataTypeStr=Inherit: Same as input  ParamDataTypeStr=Inherit: Same as input
  Gain5 : Gain  Gain=Cm_df  SaturateOnIntegerOverflow=on  OutDataTypeStr=Inherit: Same as input  ParamDataTypeStr=Inherit: Same as input
  Mux1 : Mux  Inputs=6
  Product1 : Product  SaturateOnIntegerOverflow=on  InputSameDT=on  OutDataTypeStr=Inherit: Same as first input
  Product4 : Product  SaturateOnIntegerOverflow=on  InputSameDT=on  OutDataTypeStr=Inherit: Same as first input
  Selector1 : Selector  InputPortWidth=4  Indices=4
  Sum1 : Sum  SaturateOnIntegerOverflow=on
  Sum2 : Sum  SaturateOnIntegerOverflow=on
  delCoeff : Outport
  wires:
  Selector1/1 -> Gain1/1, Product4/1, Product1/1, Gain3/1, Gain5/1
  Actuators/1 -> Selector1/1
  Gain5/1 -> Mux1/5
  Gain3/1 -> Sum2/1
  Gain4/1 -> Sum2/2
  Product1/1 -> Gain4/1
  Gain1/1 -> Sum1/1
  Gain2/1 -> Sum1/2
  Product4/1 -> Gain2/1
  Alpha/1 -> Product1/2, Product4/2
  Mux1/1 -> delCoeff/1
  Sum1/1 -> Mux1/1
  Sum2/1 -> Mux1/3
  Constant1/1 -> Mux1/2
  Constant2/1 -> Mux1/4
  Constant3/1 -> Mux1/6

== system ap_12B_cocoSim_pp/DeHavilland Beaver Airframe/Aircraft Dynamics/Total Forces  and Moments/Aerodynamics/Actuator Increments/Rudder ==
  Alpha : Inport
  Actuators : Inport  Port=2
  Constant1 : Constant  Value=0
  Constant2 : Constant  Value=0
  Gain1 : Gain  Gain=Cl_dr  SaturateOnIntegerOverflow=on  OutDataTypeStr=Inherit: Same as input  ParamDataTypeStr=Inherit: Same as input
  Gain2 : Gain  Gain=Cn_dr  SaturateOnIntegerOverflow=on  OutDataTypeStr=Inherit: Same as input  ParamDataTypeStr=Inherit: Same as input
  Gain3 : Gain  Gain=Cy_dr_alpha  SaturateOnIntegerOverflow=on  OutDataTypeStr=Inherit: Same as input  ParamDataTypeStr=Inherit: Same as input
  Gain4 : Gain  Gain=Cy_dr  SaturateOnIntegerOverflow=on  OutDataTypeStr=Inherit: Same as input  ParamDataTypeStr=Inherit: Same as input
  Gain5 : Gain  Gain=Cx_dr  SaturateOnIntegerOverflow=on  OutDataTypeStr=Inherit: Same as input  ParamDataTypeStr=Inherit: Same as input
  Mux1 : Mux  Inputs=6
  Product1 : Product  SaturateOnIntegerOverflow=on  InputSameDT=on  OutDataTypeStr=Inherit: Same as first input
  Selector1 : Selector  InputPortWidth=4  Indices=3
  Sum1 : Sum  SaturateOnIntegerOverflow=on
  delCoeff : Outport
  wires:
  Gain5/1 -> Mux1/1
  Gain4/1 -> Sum1/1
  Gain3/1 -> Sum1/2
  Gain1/1 -> Mux1/4
  Gain2/1 -> Mux1/6
  Product1/1 -> Gain3/1
  Alpha/1 -> Product1/2
  Mux1/1 -> delCoeff/1
  Actuators/1 -> Selector1/1
  Sum1/1 -> Mux1/2
  Constant1/1 -> Mux1/3
  Constant2/1 -> Mux1/5
  Selector1/1 -> Gain5/1, Gain4/1, Product1/1, Gain1/1, Gain2/1

== system ap_12B_cocoSim_pp/DeHavilland Beaver Airframe/Aircraft Dynamics/Total Forces  and Moments/Aerodynamics/Body Rate Damping/p ==
  Constant1 : Constant  Value=0
  Constant2 : Constant  Value=Cy_p
  Constant3 : Constant  Value=Cl_p
  Constant4 : Constant  Value=Cn_p
  Mux1 : Mux  Inputs=6
  delCoeff : Outport
  wires:
  Constant2/1 -> Mux1/2
  Mux1/1 -> delCoeff/1
  Constant1/1 -> Mux1/5, Mux1/3, Mux1/1
  Constant4/1 -> Mux1/6
  Constant3/1 -> Mux1/4

== system ap_12B_cocoSim_pp/DeHavilland Beaver Airframe/Aircraft Dynamics/Total Forces  and Moments/Aerodynamics/Body Rate Damping/q ==
  Constant1 : Constant  Value=0
  Constant2 : Constant  Value=Cz_q
  Constant3 : Constant  Value=Cx_q
  Constant4 : Constant  Value=Cm_q
  Constant5 : Constant  Value=Cn_q
  Mux1 : Mux  Inputs=6
  delCoeff : Outport
  wires:
  Constant2/1 -> Mux1/3
  Constant5/1 -> Mux1/6
  Constant1/1 -> Mux1/4, Mux1/2
  Constant4/1 -> Mux1/5
  Constant3/1 -> Mux1/1
  Mux1/1 -> delCoeff/1

== system ap_12B_cocoSim_pp/DeHavilland Beaver Airframe/Aircraft Dynamics/Total Forces  and Moments/Aerodynamics/Body Rate Damping/r ==
  Constant : Constant  Value=0
  Constant1 : Constant  Value=Cy_r
  Constant2 : Constant  Value=Cl_r
  Constant3 : Constant  Value=Cm_r
  Constant4 : Constant  Value=Cn_r
  Mux1 : Mux  Inputs=6
  delCoeff : Outport
  wires:
  Constant3/1 -> Mux1/5
  Constant1/1 -> Mux1/2
  Constant4/1 -> Mux1/6
  Constant2/1 -> Mux1/4
  Constant/1 -> Mux1/3, Mux1/1
  Mux1/1 -> delCoeff/1

== system ap_12B_cocoSim_pp/DeHavilland Beaver Airframe/Aircraft Dynamics/Total Forces  and Moments/Engine /pow/calc ==
  In1 : Inport
  Constant4 : Constant  Value=408.0
  Constant5 : Constant  Value=1.0
  Demux : Demux  Outputs=3
  Gain2 : Gain  Gain=0.0965  SaturateOnIntegerOverflow=on  OutDataTypeStr=Inherit: Same as input  ParamDataTypeStr=Inherit: Same as input
  Gain4 : Gain  Gain=0.8163  SaturateOnIntegerOverflow=on  OutDataTypeStr=Inherit: Same as input  ParamDataTypeStr=Inherit: Same as input
  Product2 : Product  RndMeth=Zero
  Sum1 : Sum  Inputs=+-|  SaturateOnIntegerOverflow=on
  Sum2 : Sum  Inputs=+-|  SaturateOnIntegerOverflow=on
  Terminator : Terminator
  Out1 : Outport
  wires:
  In1/1 -> Demux/1
  Product2/1 -> Out1/1
  Sum2/1 -> Product2/2
  Constant5/1 -> Sum2/1
  Gain4/1 -> Sum2/2
  Constant4/1 -> Sum1/1
  Demux/1 -> Gain2/1
  Demux/2 -> Terminator/1
  Gain2/1 -> Sum1/2
  Sum1/1 -> Product2/1
  Demux/3 -> Gain4/1

== system ap_12B_cocoSim_pp/DeHavilland Beaver Airframe/Aircraft Dynamics/Total Forces  and Moments/Engine /pow/calc1 ==
  In1 : Inport
  Constant1 : Constant  Value=2010
  Constant2 : Constant  Value=7.4
  Demux : Demux  Outputs=2
  Product1 : Product  RndMeth=Zero
  Sum3 : Sum  Inputs=++|  SaturateOnIntegerOverflow=on
  Sum4 : Sum  Inputs=|++  SaturateOnIntegerOverflow=on
  Out1 : Outport
  wires:
  In1/1 -> Demux/1
  Demux/1 -> Sum3/2
  Constant1/1 -> Sum3/1
  Sum3/1 -> Product1/1
  Demux/2 -> Sum4/1
  Constant2/1 -> Sum4/2
  Sum4/1 -> Product1/2
  Product1/1 -> Out1/1

== system ap_12B_cocoSim_pp/DeHavilland Beaver Airframe/Aircraft Dynamics/Total Forces  and Moments/Forces and Moments/Aero F&M/3x3 CrossProduct ==
  A : Inport
  B : Inport  Port=2
  A_1 : InportShadow
  B_1 : InportShadow  Port=2
  Subsystem : aerolibutil/3x3 Cross Product/Subsystem
  Subsystem1 : aerolibutil/3x3 Cross Product/Subsystem1
  Sum : Sum  Inputs=+|-  SaturateOnIntegerOverflow=on  InputSameDT=on  OutDataTypeStr=Inherit: Same as first input
  C : Outport
  wires:
  Subsystem/1 -> Sum/1
  Subsystem1/1 -> Sum/2
  B/1 -> Subsystem/2
  A/1 -> Subsystem/1
  B_1/1 -> Subsystem1/2
  A_1/1 -> Subsystem1/1
  Sum/1 -> C/1

== system ap_12B_cocoSim_pp/DeHavilland Beaver Airframe/Aircraft Dynamics/6DoF (Quaternion)/Calculate DCM & Euler Angles/Quaternions to  Direction Cosine Matrix/Quaternion Normalize/Quaternion Modulus ==
  q : Inport
  Quaternion Norm : Subsystem
  sqrt : Sqrt  AlgorithmType=Newton-Raphson  SaturateOnIntegerOverflow=on
  |q| : Outport
  wires:
  Quaternion Norm/1(norm(q)) -> sqrt/1
  sqrt/1 -> |q|/1
  q/1 -> Quaternion Norm/1(q)

== system ap_12B_cocoSim_pp/DeHavilland Beaver Airframe/Aircraft Dynamics/6DoF (Quaternion)/Calculate DCM & Euler Angles/Quaternions to Rotation Angles (ZYX)/Quaternion Normalize/Quaternion Modulus ==
  q : Inport
  Quaternion Norm : Subsystem
  sqrt : Sqrt  AlgorithmType=Newton-Raphson  SaturateOnIntegerOverflow=on
  |q| : Outport
  wires:
  Quaternion Norm/1(norm(q)) -> sqrt/1
  sqrt/1 -> |q|/1
  q/1 -> Quaternion Norm/1(q)

== system ap_12B_cocoSim_pp/DeHavilland Beaver Airframe/Aircraft Dynamics/6DoF (Quaternion)/Calculate DCM & Euler Angles/Quaternions to  Direction Cosine Matrix/Quaternion Normalize/Quaternion Modulus/Quaternion Norm ==
  q : Inport
  Demux : Demux
  Product{,1..3} (4 alike) : Product
  Sum : Sum  Inputs=4
  norm(q) : Outport
  wires:
  Demux/2 -> Product1/2, Product1/1
  q/1 -> Demux/1
  Sum/1 -> norm(q)/1
  Demux/1 -> Product/2, Product/1
  Product3/1 -> Sum/4
  Demux/3 -> Product2/2, Product2/1
  Product2/1 -> Sum/3
  Product/1 -> Sum/1
  Product1/1 -> Sum/2
  Demux/4 -> Product3/2, Product3/1

== system ap_12B_cocoSim_pp/DeHavilland Beaver Airframe/Aircraft Dynamics/6DoF (Quaternion)/Calculate DCM & Euler Angles/Quaternions to Rotation Angles (ZYX)/Quaternion Normalize/Quaternion Modulus/Quaternion Norm ==
  q : Inport
  Demux : Demux
  Product{,1..3} (4 alike) : Product
  Sum : Sum  Inputs=4
  norm(q) : Outport
  wires:
  Demux/2 -> Product1/2, Product1/1
  q/1 -> Demux/1
  Sum/1 -> norm(q)/1
  Demux/1 -> Product/2, Product/1
  Product3/1 -> Sum/4
  Demux/3 -> Product2/2, Product2/1
  Product2/1 -> Sum/3
  Product/1 -> Sum/1
  Product1/1 -> Sum/2
  Demux/4 -> Product3/2, Product3/1
